simulink model "booster_control"  (R2024b)
settings: Solver=VariableStepAuto  StartTime=0.0  StopTime=Tfin_cont  RelTol=1e-3
values from neighbouring files (symbols this model uses):
  a = pi*r^2    (= 78.5398163397)    [script_project.m]
  Cd = 1.2    [script_project.m]
  g = 9.81    [script_project.m]
  h = 70    [script_project.m]
  J = (1/12)*m*(b^2 + h^2)    (= 208333333.333)    [script_project.m]
  K = -place(A, B, desired_poles)    [script_project.m]
  m = 500000    [script_project.m]
  rho = 1.225    [script_project.m]
  u0 = [u1eq u2eq u3eq]'    [script_project.m]
  z0 = [x2eq x2doteq thetaeq thetadoteq]'    [script_project.m]
  z0_cont = z0 + dz0_cont    [script_project.m]
undefined symbols (not defined in the file or in its folder): A, B
settings Model: Creator=martinhaugen  LastModifiedBy=martinhaugen

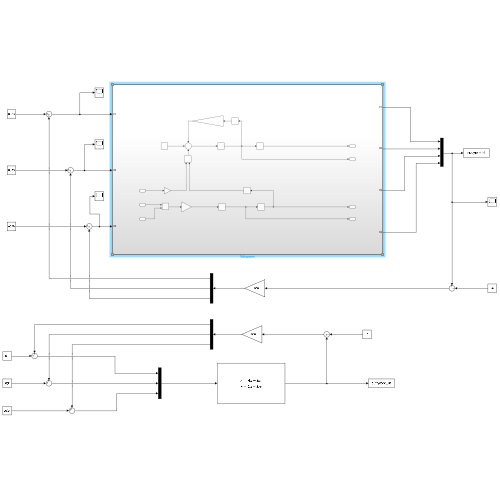
[thumbnail: Simulink's stored preview of the top-level diagram]
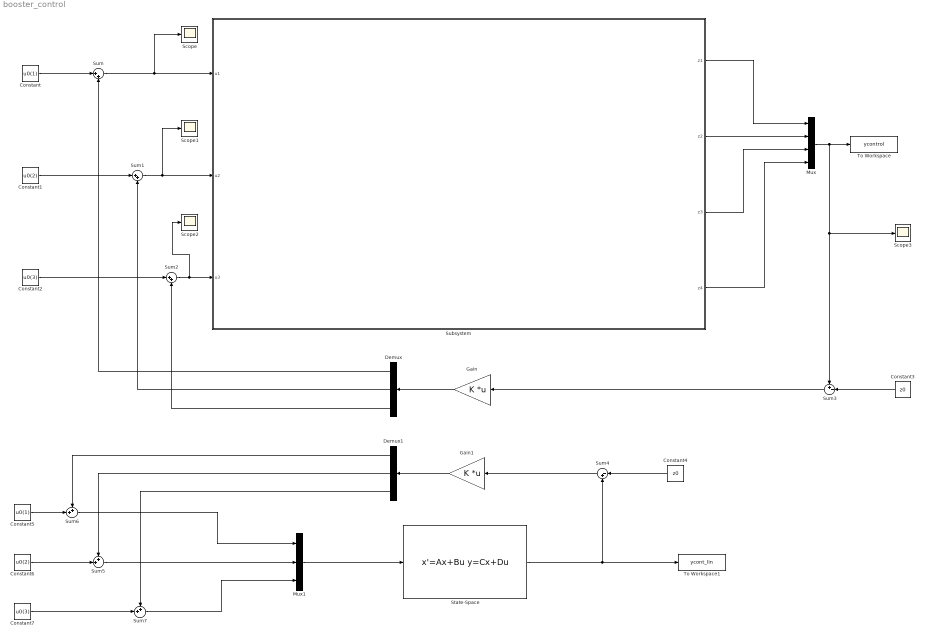
== system booster_control ==
  Constant : Constant  Value=u0(1)
  Constant1 : Constant  Value=u0(2)
  Constant2 : Constant  Value=u0(3)
  Constant3 : Constant  Value=z0
  Constant4 : Constant  Value=z0
  Constant5 : Constant  Value=u0(1)
  Constant6 : Constant  Value=u0(2)
  Constant7 : Constant  Value=u0(3)
  Demux : Demux  Outputs=3
  Demux1 : Demux  Outputs=3
  Gain : Gain  Gain=K  Multiplication=Matrix(K*u)
  Gain1 : Gain  Gain=K  Multiplication=Matrix(K*u)
  Mux : Mux
  Mux1 : Mux  Inputs=3
  Scope{,1..3} (4 alike) : Scope
  State-Space : StateSpace  A=A  B=B  C=[1 0 0 0; 0 1 0 0; 0 0 1 0; 0 0 0 1]  D=[0 0 0; 0 0 0; 0 0 0; 0 0 0]  InitialCondition=z0_cont
  Subsystem : Subsystem
  Sum : Sum  Inputs=|++
  Sum1 : Sum  Inputs=|++
  Sum2 : Sum  Inputs=|++
  Sum3 : Sum  Inputs=+-|
  Sum4 : Sum  Inputs=|-+
  Sum5 : Sum  Inputs=++|
  Sum6 : Sum  Inputs=++|
  Sum7 : Sum  Inputs=++|
  To Workspace : ToWorkspace  VariableName=ycontrol  SaveFormat=Timeseries  SampleTime=-1
  To Workspace1 : ToWorkspace  VariableName=ycont_lin  SaveFormat=Timeseries  SampleTime=-1
  wires:
  Subsystem/1(z1) -> Mux/1
  Mux/1 -> To Workspace/1, Sum3/1, Scope3/1
  Subsystem/2(z2) -> Mux/2
  Subsystem/3(z3) -> Mux/3
  Subsystem/4(z4) -> Mux/4
  Gain/1 -> Demux/1
  Demux/1 -> Sum/2
  Constant/1 -> Sum/1
  Sum/1 -> Scope/1, Subsystem/1(u1)
  Constant1/1 -> Sum1/1
  Demux/2 -> Sum1/2
  Sum1/1 -> Scope1/1, Subsystem/2(u2)
  Constant2/1 -> Sum2/1
  Sum2/1 -> Subsystem/3(u3), Scope2/1
  Demux/3 -> Sum2/2
  Sum3/1 -> Gain/1
  Constant3/1 -> Sum3/2
  Mux1/1 -> State-Space/1
  State-Space/1 -> To Workspace1/1, Sum4/2
  Gain1/1 -> Demux1/1
  Demux1/1 -> Sum6/1
  Demux1/2 -> Sum5/1
  Demux1/3 -> Sum7/1
  Constant5/1 -> Sum6/2
  Constant6/1 -> Sum5/2
  Constant7/1 -> Sum7/2
  Sum6/1 -> Mux1/1
  Sum5/1 -> Mux1/2
  Sum7/1 -> Mux1/3
  Sum4/1 -> Gain1/1
  Constant4/1 -> Sum4/1

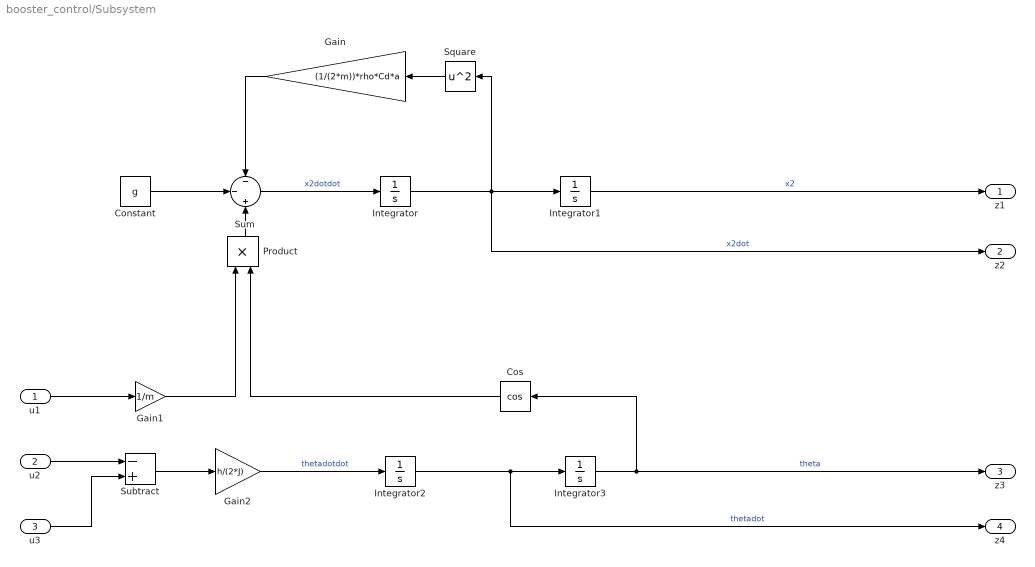
== system booster_control/Subsystem ==
  u1 : Inport
  u2 : Inport  Port=2
  u3 : Inport  Port=3
  Constant : Constant  Value=g
  Cos : Trigonometry  Operator=cos
  Gain : Gain  Gain=(1/(2*m))*rho*Cd*a
  Gain1 : Gain  Gain=1/m
  Gain2 : Gain  Gain=h/(2*J)
  Integrator : Integrator  InitialCondition=z0_cont(2)  ContinuousStateAttributes='z2'
  Integrator1 : Integrator  InitialCondition=z0_cont(1)  ContinuousStateAttributes='z1'
  Integrator2 : Integrator  InitialCondition=z0_cont(4)  ContinuousStateAttributes='z4'
  Integrator3 : Integrator  InitialCondition=z0_cont(3)  ContinuousStateAttributes='z3'
  Product : Product
  Square : Math  Operator=square
  Subtract : Sum  Inputs=-+
  Sum : Sum  Inputs=-|-|+
  z1 : Outport
  z2 : Outport  Port=2
  z3 : Outport  Port=3
  z4 : Outport  Port=4
  wires:
  u2/1 -> Subtract/1
  Constant/1 -> Sum/2
  Square/1 -> Gain/1
  Product/1 -> Sum/3
  Subtract/1 -> Gain2/1
  Integrator/1 -> z2/1, Integrator1/1, Square/1  "x2dot"
  Gain2/1 -> Integrator2/1  "thetadotdot"
  Cos/1 -> Product/2
  u3/1 -> Subtract/2
  Integrator2/1 -> z4/1, Integrator3/1  "thetadot"
  u1/1 -> Gain1/1
  Gain/1 -> Sum/1
  Sum/1 -> Integrator/1  "x2dotdot"
  Gain1/1 -> Product/1
  Integrator3/1 -> z3/1, Cos/1  "theta"
  Integrator1/1 -> z1/1  "x2"
